simulink model "SVPWM_INVERTER"  (R2022a)
settings: Solver=VariableStepAuto  StartTime=0.0  StopTime=0.8  RelTol=1e-3
libraries: spsMosfetLib x6, spsThreePhaseSeriesRLCBranchLib x3, spsThreePhaseVIMeasurementLib x2, spsDCVoltageSourceLib x1, spsGroundLib x1, spspowerguiLib x1, spsFundamentalPLLDrivenLib x1, spsPLLLib x1, simulink x1
settings Model: Creator=Abdo  LastModifiedBy=Abdo
settings ModelReferenceCC: EnableRefExpFcnMdlSchedulingChecks=off
settings RTWCC: Description=Generic Real-Time Target  GPUComputeCapability=5.0

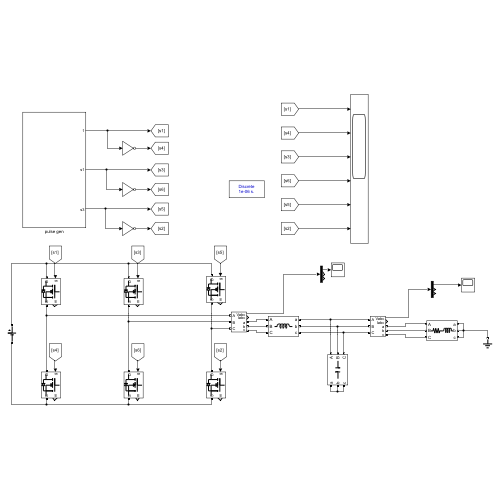
[thumbnail: Simulink's stored preview of the top-level diagram]
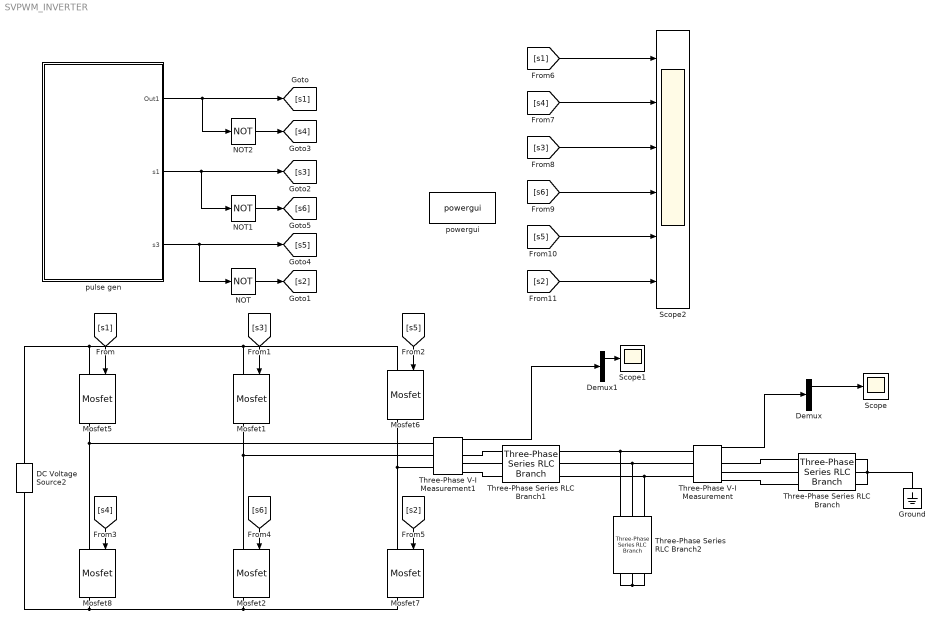
== system SVPWM_INVERTER ==
  DC Voltage Source2 : spsDCVoltageSourceLib/DC Voltage Source  Amplitude=320  Measurements=None
  Demux : Demux  Outputs=3
  Demux1 : Demux  Outputs=3
  Ground : spsGroundLib/Ground  LConnTagsString=a
  Mosfet{1..2,5..8} (6 alike) : spsMosfetLib/Mosfet  Ron=0.1  Lon=0  Rd=0.01  Vfd=0  IC=0  Rs=1e5  Cs=inf  Measurements=on
  NOT : Logic  Operator=NOT  IconShape=distinctive  AllPortsSameDT=off  OutDataTypeStr=boolean
  NOT1 : Logic  Operator=NOT  IconShape=distinctive  AllPortsSameDT=off  OutDataTypeStr=boolean
  NOT2 : Logic  Operator=NOT  IconShape=distinctive  AllPortsSameDT=off  OutDataTypeStr=boolean
  Scope : Scope
  Scope1 : Scope
  Scope2 : Scope  NumInputPorts=6
  Three-Phase Series RLC Branch : spsThreePhaseSeriesRLCBranchLib/Three-Phase Series RLC Branch  LConnTagsString=A|B|C  RConnTagsString=A|B|C  BranchType=RL  Resistance=1  Inductance=1e-3  Capacitance=1e-6  Measurements=None
  Three-Phase Series RLC Branch1 : spsThreePhaseSeriesRLCBranchLib/Three-Phase Series RLC Branch  LConnTagsString=A|B|C  RConnTagsString=A|B|C  BranchType=L  Resistance=1  Inductance=50e-3  Capacitance=1e-6  Measurements=None
  Three-Phase Series RLC Branch2 : spsThreePhaseSeriesRLCBranchLib/Three-Phase Series RLC Branch  LConnTagsString=A|B|C  RConnTagsString=A|B|C  BranchType=C  Resistance=1  Inductance=1e-3  Capacitance=100e-4  Measurements=None
  Three-Phase V-I Measurement : spsThreePhaseVIMeasurementLib/Three-Phase V-I Measurement  VoltageMeasurement=phase-to-ground  SetLabelV=off  LabelV=Vabc  Vpu=off  VpuLL=off  CurrentMeasurement=yes  SetLabelI=off  LabelI=Iabc  Ipu=off  Pbase=100e6  Vbase=500e3  OutputType=Complex  PhasorSimulation=off  PSBequivalent=0
  Three-Phase V-I Measurement1 : spsThreePhaseVIMeasurementLib/Three-Phase V-I Measurement  VoltageMeasurement=phase-to-ground  SetLabelV=off  LabelV=Vabc  Vpu=off  VpuLL=off  CurrentMeasurement=yes  SetLabelI=off  LabelI=Iabc  Ipu=off  Pbase=100e6  Vbase=500e3  OutputType=Complex  PhasorSimulation=off  PSBequivalent=0
  powergui : spspowerguiLib/powergui  Priority=1  SimulationMode=Discrete  SampleTime=1e-6  frequency=60  Iterations=50  frequencyindice=0  Pbase=100e6  ErrMax=1e-4  UnitsV=kV  UnitsW=MW  buscounter=0  FunctionMessages=off  echomessages=off  EnableUseOfTLC=off  CurrentSourceSwitches=off  DisableSnubberDevices=off  DisableRonSwitches=off  DisableVfSwitches=off  DisplayEquations=off  AutomaticDiscreteSolvers=off  SolverType=Tustin/Backward Euler (TBE)  Interpol=off  ExternalGateDelay=off  methode=off  Ts=100  x0status=blocks  SPID=on  SwTol=0  HookPort=off  NonlinearTolerance=1e-4  nMaxIteration=100  ContinueOnMaxIteration=off  RestoreLinks=warning  ResistiveCurrentMeasurement=off  Frange=[0:2:500]  Ylog=off  Xlog=on  ShowGrid=off  save=off  variable=ZData  structure=0  ZoomFFT=off  StartTime=0.0  cycles=1  DisplayStyle=1  fundamental=60  FreqAxis=off  MaxFrequency=1000  frequencyindicesteady=1  RmsSteady=1  display=off
  pulse gen : Subsystem
  wires:
  [s1] -> Mosfet5/1
  [s3] -> Mosfet1/1
  [s5] -> Mosfet6/1
  [s4] -> Mosfet8/1
  [s6] -> Mosfet2/1
  [s2] -> Mosfet7/1
  NOT/1 -> [s2]
  NOT1/1 -> [s6]
  NOT2/1 -> [s4]
  pulse gen/1(Out1) -> NOT2/1, [s1]
  pulse gen/2(s1) -> [s3], NOT1/1
  pulse gen/3(s3) -> NOT/1, [s5]
  Three-Phase V-I Measurement/1 -> Demux/1
  Demux/1 -> Scope/1
  Demux1/1 -> Scope1/1
  Three-Phase V-I Measurement1/1 -> Demux1/1
  [s1] -> Scope2/1
  [s4] -> Scope2/2
  [s3] -> Scope2/3
  [s6] -> Scope2/4
  [s5] -> Scope2/5
  [s2] -> Scope2/6
  connections:
  Mosfet7/LConn1 -- Three-Phase V-I Measurement1/LConn3 -- Mosfet6/RConn1
  Mosfet2/LConn1 -- Three-Phase V-I Measurement1/LConn2 -- Mosfet1/RConn1
  Mosfet8/LConn1 -- Three-Phase V-I Measurement1/LConn1 -- Mosfet5/RConn1
  Mosfet8/RConn1 -- DC Voltage Source2/LConn1 -- Mosfet2/RConn1 -- Mosfet7/RConn1
  Mosfet6/LConn1 -- Mosfet5/LConn1 -- DC Voltage Source2/RConn1 -- Mosfet1/LConn1
  Three-Phase Series RLC Branch/RConn1 -- Ground/LConn1 -- Three-Phase Series RLC Branch/RConn3 -- Three-Phase Series RLC Branch/RConn2
  Three-Phase Series RLC Branch1/RConn1 -- Three-Phase Series RLC Branch2/LConn1 -- Three-Phase V-I Measurement/LConn1
  Three-Phase Series RLC Branch2/LConn2 -- Three-Phase V-I Measurement/LConn2 -- Three-Phase Series RLC Branch1/RConn2
  Three-Phase Series RLC Branch2/LConn3 -- Three-Phase V-I Measurement/LConn3 -- Three-Phase Series RLC Branch1/RConn3
  Three-Phase Series RLC Branch2/RConn1 -- Three-Phase Series RLC Branch2/RConn2 -- Three-Phase Series RLC Branch2/RConn3
  Three-Phase Series RLC Branch/LConn1 -- Three-Phase V-I Measurement/RConn1
  Three-Phase V-I Measurement/RConn2 -- Three-Phase Series RLC Branch/LConn2
  Three-Phase Series RLC Branch/LConn3 -- Three-Phase V-I Measurement/RConn3
  Three-Phase V-I Measurement1/RConn1 -- Three-Phase Series RLC Branch1/LConn1
  Three-Phase V-I Measurement1/RConn2 -- Three-Phase Series RLC Branch1/LConn2
  Three-Phase V-I Measurement1/RConn3 -- Three-Phase Series RLC Branch1/LConn3

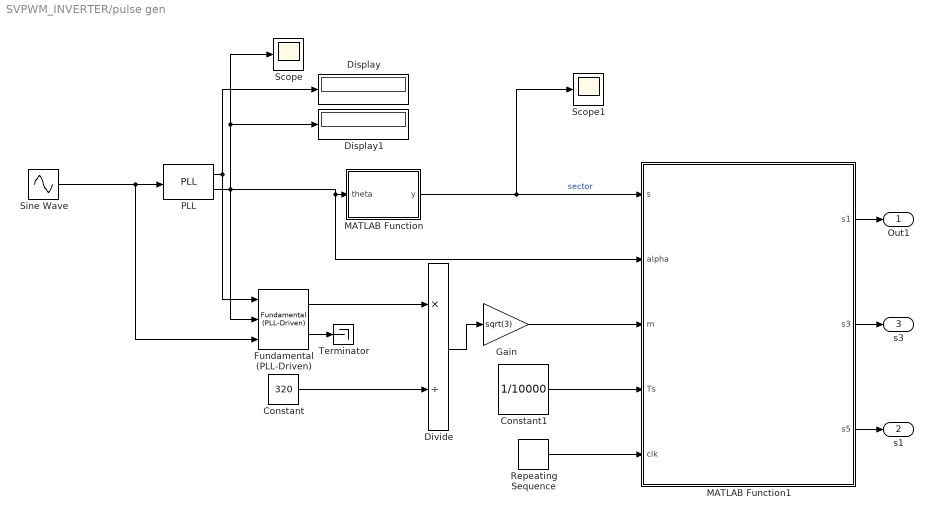
== system SVPWM_INVERTER/pulse gen ==
  Constant : Constant  Value=320
  Constant1 : Constant  Value=1/10000
  Display : Display
  Display1 : Display
  Divide : Product  Inputs=*/
  Fundamental (PLL-Driven) : spsFundamentalPLLDrivenLib/Fundamental (PLL-Driven)  Finit=60  Fmin=45  InInit=[1, 0]  Ts=0
  Gain : Gain  Gain=sqrt(3)
  MATLAB Function : MATLAB Function  TreatAsAtomicUnit=on
  MATLAB Function1 : MATLAB Function  TreatAsAtomicUnit=on
  PLL : spsPLLLib/PLL  Fmin=45  Par_Init=[0, 60]  ParK=[180, 3200, 1]  TcD=1e-4  MaxRateChangeFreq=12  FilterCutOffFreq=25  Ts=0  AGC=on
  Repeating Sequence : simulink/Sources/Repeating Sequence  rep_seq_t=[0 1/10000]  rep_seq_y=[0 1/10000]
  Scope : Scope
  Scope1 : Scope
  Sine Wave : Sin  Amplitude=220*sqrt(2)  Frequency=100*pi  SampleTime=0
  Terminator : Terminator
  Out1 : Outport
  s1 : Outport  Port=2
  s3 : Outport  Port=3
  wires:
  Sine Wave/1 -> Fundamental (PLL-Driven)/3, PLL/1
  PLL/1 -> Display/1, Fundamental (PLL-Driven)/1
  PLL/2 -> Scope/1, Display1/1, Fundamental (PLL-Driven)/2, MATLAB Function1/2(alpha), MATLAB Function/1(theta)
  MATLAB Function/1(y) -> Scope1/1, MATLAB Function1/1(s)  "sector"
  Fundamental (PLL-Driven)/2 -> Terminator/1
  Fundamental (PLL-Driven)/1 -> Divide/1
  Constant/1 -> Divide/2
  Divide/1 -> Gain/1
  Gain/1 -> MATLAB Function1/3(m)
  Constant1/1 -> MATLAB Function1/4(Ts)
  Repeating Sequence/1 -> MATLAB Function1/5(clk)
  MATLAB Function1/1(s1) -> Out1/1
  MATLAB Function1/3(s5) -> s1/1
  MATLAB Function1/2(s3) -> s3/1

== matlab function SVPWM_INVERTER/pulse gen/MATLAB Function1 ==
  data: s1 output; s3 output; s input; alpha input; m input; Ts input; clk input; s5 output
function [s1,s3,s5] = fcn(s,alpha,m,Ts,clk)

T1 = Ts*m*sin((pi/3)-(alpha-(pi/3)*(s-1)));
T2 = Ts*m*sin(alpha-(pi/3)*(s-1));
T0 = Ts - T1 - T2;

switch(s)
    case (1)
        if( clk >= T0/4 && clk < (T1 + T2 + T0*3/4) )
            s1 = 1;
        else
            s1 = 0;
        end 
        if( clk >= (T0/4 + T1/2) && clk < (T0*3/4 + T1/2 + T2) )
            s3 = 1;
        else
            s3 = 0;
        end 
        if( clk >= (T0/4 + T1/2 + T2/2) && clk < (T0*3/4 + T1/2 + T2/2) )
            s5 = 1;
        else
            s5 = 0;
        end 
    case (2)
        if( clk >= (T0/4 + T1/2) && clk < (T0*3/4 + T1/2 + T2) )
            s1 = 1;
        else
            s1 = 0;
        end 
        if( clk >= T0/4 && clk < (T1 + T2 + T0*3/4) )
            s3 = 1;
        else
            s3 = 0;
        end 
        if( clk >= (T0/4 + T1/2 + T2/2) && clk < (T0*3/4 + T1/2 + T2/2) )
            s5 = 1;
        else
            s5 = 0;
        end 
    case (3)
         if( clk >= (T0/4 + T1/2 + T2/2) && clk < (T0*3/4 + T1/2 + T2/2) )
            s1 = 1;
        else
            s1 = 0;
        end 
        if( clk >= T0/4 && clk < (T1 + T2 + T0*3/4) )
            s3 = 1;
        else
            s3 = 0;
        end 
        if( clk >= (T0/4 + T1/2) && clk < (T0*3/4 + T1/2 + T2) )
            s5 = 1;
        else
            s5 = 0;
        end 
    case (4)
        if( clk >= (T0/4 + T1/2 + T2/2) && clk < (T0*3/4 + T1/2 + T2/2) )
            s1 = 1;
        else
            s1 = 0;
        end 
        if( clk >= (T0/4 + T1/2) && clk < (T0*3/4 + T1/2 + T2) )
            s3 = 1;
        else
            s3 = 0;
        end 
        if( clk >= T0/4 && clk < (T1 + T2 + T0*3/4) )
            s5 = 1;
        else
            s5 = 0;
        end 
    case (5)
        if( clk >= (T0/4 + T1/2) && clk < (T0*3/4 + T1/2 + T2) )
            s1 = 1;
        else
            s1 = 0;
        end 
        if( clk >= (T0/4 + T1/2 + T2/2) && clk < (T0*3/4 + T1/2 + T2/2) )
            s3 = 1;
        else
            s3 = 0;
        end 
        if( clk >= T0/4 && clk < (T1 + T2 + T0*3/4) )
            s5 = 1;
        else
            s5 = 0;
        end 
    case (6)
        if( clk >= T0/4 && clk < (T1 + T2 + T0*3/4) )
            s1 = 1;
        else
            s1 = 0;
        end 
        if( clk >= (T0/4 + T1/2 + T2/2) && clk < (T0*3/4 + T1/2 + T2/2) )
            s3 = 1;
        else
            s3 = 0;
        end 
        if( clk >= (T0/4 + T1/2) && clk < (T0*3/4 + T1/2 + T2) )
            s5 = 1;
        else
            s5 = 0;
        end 
    otherwise
        s1 = 0;
        s3 = 0;
        s5 = 0;
end

== matlab function SVPWM_INVERTER/pulse gen/MATLAB Function ==
  data: theta input; y output
function y = fcn(theta)
if (theta >= 0 && theta <= pi/3)
    u = 1;
elseif (theta >= pi/3 && theta <= 2*pi/3)
    u = 2;
elseif (theta >= 2*pi/3 && theta <= pi)
    u = 3;
elseif (theta >= pi && theta <= 4*pi/3)
    u = 4;
elseif (theta >= 4*pi/3 && theta <= 5*pi/3)
    u = 5;
else
    u = 6;
end
y = u;
